simulink model "Bus"  (Simulink 7.4)
settings: Solver=ode45  StartTime=0.0  StopTime=10.0  RelTol=1e-3
PostLoadFcn:
  | load Bus.mat
settings Model: Creator=dread  LastModifiedBy=dread

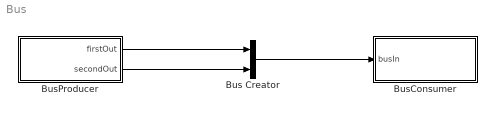
== system Bus ==
  Bus Creator : BusCreator  Inputs=2  UseBusObject=on
      settings: BusObject=Bus
  BusConsumer : Subsystem
  BusProducer : Subsystem
  wires:
  BusProducer/1(firstOut) -> Bus Creator/1
  BusProducer/2(secondOut) -> Bus Creator/2
  Bus Creator/1 -> BusConsumer/1(busIn)

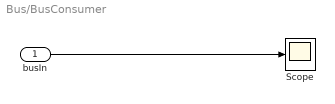
== system Bus/BusConsumer ==
  busIn : Inport  UseBusObject=on  OutDataType=fixdt(1, 16)  OutScaling=2^0
      settings: BusObject=Bus
  Scope : Scope
  wires:
  busIn/1 -> Scope/1

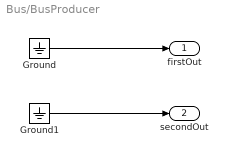
== system Bus/BusProducer ==
  Ground : Ground
  Ground1 : Ground
  firstOut : Outport  OutDataType=fixdt(1, 16)  OutScaling=2^0
  secondOut : Outport  Port=2  OutDataType=fixdt(1, 16)  OutScaling=2^0
  wires:
  Ground1/1 -> secondOut/1
  Ground/1 -> firstOut/1
